simulink model "q_sip_lqr_mq3_ip01"  (Simulink 4.00)
settings: Solver=ode4  SolverMode=SingleTasking  StartTime=0.0  StopTime=9999  FixedStep=0.001  RelTol=1e-3  AbsTol=1e-6
values from neighbouring files (symbols this model uses):
  C = eye( 4 )    [d_ip01_2_sip_lqr.m]
  D = zeros( 4, 1 )    [d_ip01_2_sip_lqr.m]
undefined symbols (not defined in the file or in its folder): A, ALPHA_LIM_ENABLE, ALPHA_MAX, ALPHA_MIN, B, K, K_CABLE, K_PC, K_PP, simget, VMAX_DAC, VMAX_UPM, wcf, X_LIM_ENABLE, X_MAX, X_MIN, zetaf
libraries: qctools x6, simulink_extras x3
settings Model: LastModifiedBy=herve  LimitDataPoints=off  SimulationMode=external  RTWSystemTargetFile=wincon.tlc  RTWTemplateMakefile=nt_msvc.tmf  RTWMakeCommand=make_wc  ExtModeMexFile=wc_comm  ExtModeArmWhenConnect=off  OptimizeBlockIOStorage=off

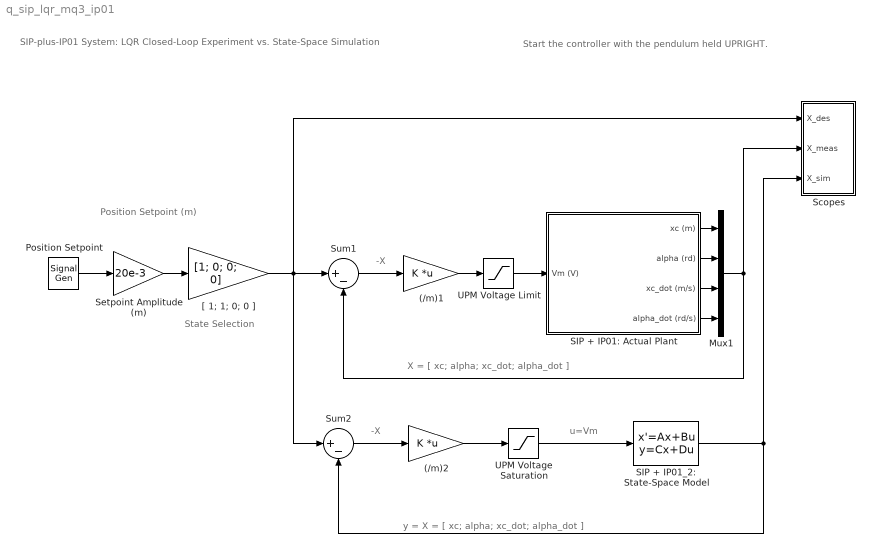
== system q_sip_lqr_mq3_ip01 ==
  note: SIP-plus-IP01 System: LQR Closed-Loop
      | Experiment vs. State-Space Simulation
  note: u=Vm
  note: X = [ xc; alpha; xc_dot; alpha_dot ]
  note: -X
  note: -X
  note: State Selection
  note: Start the controller with the pendulum held UPRIGHT.
  note: Position Setpoint (m)
  note: y = X = [ xc; alpha; xc_dot; alpha_dot ]
  (/m)1 : Gain  Gain=K  Multiplication=Matrix(K*u)  SaturateOnIntegerOverflow=on
  (/m)2 : Gain  Gain=K  Multiplication=Matrix(K*u)  SaturateOnIntegerOverflow=on
  Mux1 : Mux  Inputs=4
  Position Setpoint : SignalGenerator  WaveForm=square  Amplitude=1  Frequency=0.2  Units=Hertz
  SIP + IP01: Actual Plant : Subsystem
      settings: RTWFcnNameOpts=Auto  RTWFileNameOpts=Auto
  SIP + IP01_2: State-Space Model : StateSpace  A=A  B=B  C=C  D=D  X0=0  AbsoluteTolerance=auto  Realization=auto
  Scopes : Subsystem
      settings: RTWFcnNameOpts=Auto  RTWFileNameOpts=Auto
  Setpoint Amplitude (m) : Gain  Gain=20e-3  Multiplication=Element-wise(K.*u)  SaturateOnIntegerOverflow=on
  Sum1 : Sum  Inputs=|+-  SaturateOnIntegerOverflow=on
  Sum2 : Sum  Inputs=|+-  SaturateOnIntegerOverflow=on
  UPM Voltage Limit : Saturate  UpperLimit=VMAX_UPM  LowerLimit=- VMAX_UPM  LinearizeAsGain=on
  UPM Voltage Saturation : Saturate  UpperLimit=VMAX_UPM  LowerLimit=- VMAX_UPM  LinearizeAsGain=on
  "[ 1; 1; 0; 0 ]" : Gain  Gain=[1; 0; 0; 0]  Multiplication=Element-wise(K.*u)  SaturateOnIntegerOverflow=on
  wires:
  UPM Voltage Limit/1 -> SIP + IP01: Actual Plant/1(Vm (V))
  SIP + IP01: Actual Plant/1(xc (m)) -> Mux1/1
  (/m)1/1 -> UPM Voltage Limit/1
  SIP + IP01: Actual Plant/2(alpha (rd)) -> Mux1/2
  SIP + IP01: Actual Plant/4(alpha_dot (rd/s)) -> Mux1/4
  UPM Voltage Saturation/1 -> SIP + IP01_2: State-Space Model/1
  (/m)2/1 -> UPM Voltage Saturation/1
  Sum2/1 -> (/m)2/1
  Sum1/1 -> (/m)1/1
  "[ 1; 1; 0; 0 ]"/1 -> Sum1/1, Sum2/1, Scopes/1(X_des)
  Mux1/1 -> Sum1/2, Scopes/2(X_meas)
  SIP + IP01_2: State-Space Model/1 -> Sum2/2, Scopes/3(X_sim)
  Setpoint Amplitude (m)/1 -> "[ 1; 1; 0; 0 ]"/1
  SIP + IP01: Actual Plant/3(xc_dot (m/s)) -> Mux1/3
  Position Setpoint/1 -> Setpoint Amplitude (m)/1

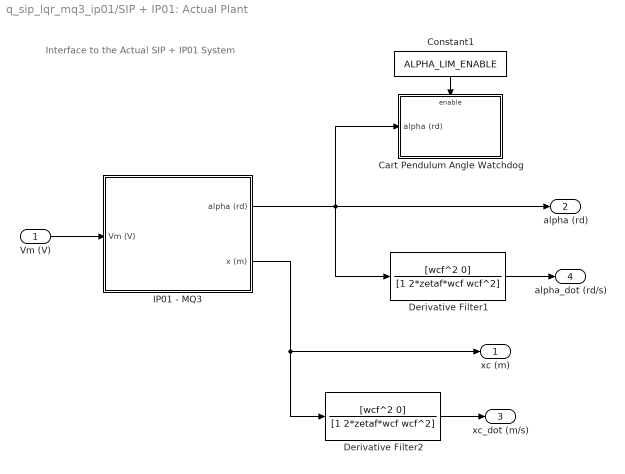
== system q_sip_lqr_mq3_ip01/SIP + IP01: Actual Plant ==
  note: Interface to the Actual
      | SIP + IP01 System
  Vm (V) : Inport  Port=1  LatchInput=off
  Cart Pendulum Angle Watchdog : Subsystem  TreatAsAtomicUnit=on
      settings: RTWFcnNameOpts=Auto  RTWFileNameOpts=Auto
  Constant1 : Constant  Orientation=down  Value=ALPHA_LIM_ENABLE
  Derivative Filter1 : TransferFcn  Numerator=[wcf^2 0]  Denominator=[1 2*zetaf*wcf wcf^2]  AbsoluteTolerance=auto  Realization=auto
  Derivative Filter2 : TransferFcn  Numerator=[wcf^2 0]  Denominator=[1 2*zetaf*wcf wcf^2]  AbsoluteTolerance=auto  Realization=auto
  IP01 - MQ3 : Subsystem
      settings: RTWFcnNameOpts=Auto  RTWFileNameOpts=Auto
  xc (m) : Outport  Port=1  InitialOutput=0
  alpha (rd) : Outport  Port=2  InitialOutput=0
  xc_dot (m/s) : Outport  Port=3  InitialOutput=0
  alpha_dot (rd/s) : Outport  Port=4  InitialOutput=0
  wires:
  Vm (V)/1 -> IP01 - MQ3/1(Vm (V))
  IP01 - MQ3/2(x (m)) -> Derivative Filter2/1, xc (m)/1
  IP01 - MQ3/1(alpha (rd)) -> Derivative Filter1/1, alpha (rd)/1, Cart Pendulum Angle Watchdog/1(alpha (rd))
  Derivative Filter2/1 -> xc_dot (m/s)/1
  Derivative Filter1/1 -> alpha_dot (rd/s)/1
  Constant1/1 -> Cart Pendulum Angle Watchdog/Enable

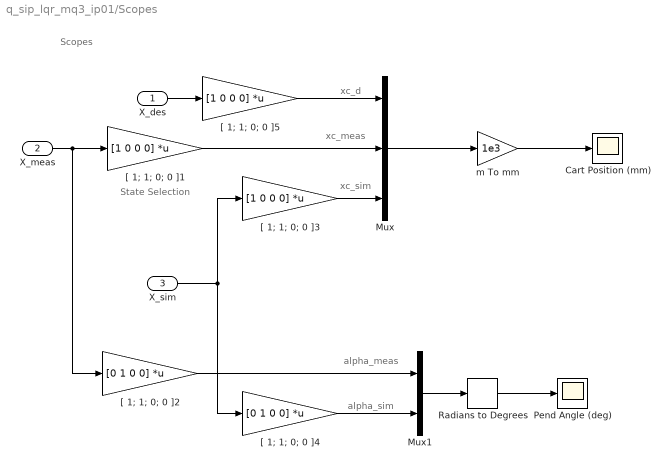
== system q_sip_lqr_mq3_ip01/Scopes ==
  note: xc_meas
  note: State Selection
  note: alpha_meas
  note: alpha_sim
  note: xc_sim
  note: xc_d
  note: Scopes
  X_des : Inport  Port=1  LatchInput=off
  X_meas : Inport  Port=2  LatchInput=off
  X_sim : Inport  Port=3  LatchInput=off
  Cart Position (mm) : Scope
      settings: TickLabels=on  TimeRange=1.000000  YMin=-250  YMax=250  SaveToWorkspace=off  DataFormat=Array  LimitDataPoints=on  MaxDataPoints=5000
  Mux : Mux  Inputs=3
  Mux1 : Mux  Inputs=2
  Pend Angle (deg) : Scope
      settings: TickLabels=on  TimeRange=1.000000  YMin=-250  YMax=250  SaveToWorkspace=off  SaveName=ScopeData  DataFormat=Array  LimitDataPoints=on  MaxDataPoints=5000
  Radians to Degrees : simulink_extras/Transformations/Radians to Degrees
  "[ 1; 1; 0; 0 ]1" : Gain  Gain=[1 0 0 0]  Multiplication=Matrix(K*u)  SaturateOnIntegerOverflow=on
  "[ 1; 1; 0; 0 ]2" : Gain  Gain=[0 1 0 0]  Multiplication=Matrix(K*u)  SaturateOnIntegerOverflow=on
  "[ 1; 1; 0; 0 ]3" : Gain  Gain=[1 0 0 0]  Multiplication=Matrix(K*u)  SaturateOnIntegerOverflow=on
  "[ 1; 1; 0; 0 ]4" : Gain  Gain=[0 1 0 0]  Multiplication=Matrix(K*u)  SaturateOnIntegerOverflow=on
  "[ 1; 1; 0; 0 ]5" : Gain  Gain=[1 0 0 0]  Multiplication=Matrix(K*u)  SaturateOnIntegerOverflow=on
  m To mm : Gain  Gain=1e3  Multiplication=Element-wise(K.*u)  SaturateOnIntegerOverflow=on
  wires:
  Mux/1 -> m To mm/1
  m To mm/1 -> Cart Position (mm)/1
  "[ 1; 1; 0; 0 ]1"/1 -> Mux/2
  X_des/1 -> "[ 1; 1; 0; 0 ]5"/1
  X_meas/1 -> "[ 1; 1; 0; 0 ]1"/1, "[ 1; 1; 0; 0 ]2"/1
  Mux1/1 -> Radians to Degrees/1
  Radians to Degrees/1 -> Pend Angle (deg)/1
  X_sim/1 -> "[ 1; 1; 0; 0 ]3"/1, "[ 1; 1; 0; 0 ]4"/1
  "[ 1; 1; 0; 0 ]3"/1 -> Mux/3
  "[ 1; 1; 0; 0 ]5"/1 -> Mux/1
  "[ 1; 1; 0; 0 ]2"/1 -> Mux1/1
  "[ 1; 1; 0; 0 ]4"/1 -> Mux1/2

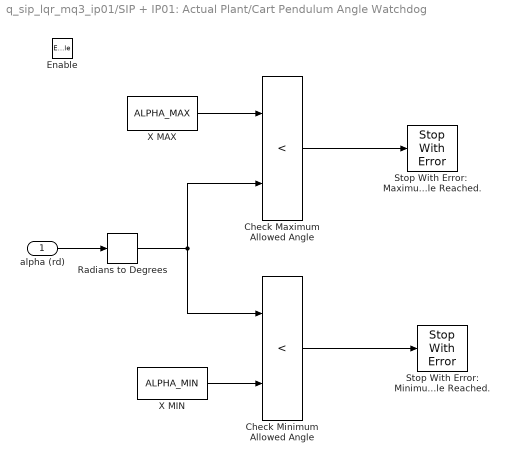
== system q_sip_lqr_mq3_ip01/SIP + IP01: Actual Plant/Cart Pendulum Angle Watchdog ==
  alpha (rd) : Inport  Port=1  LatchInput=off
  Enable : EnablePort
  Check Maximum Allowed Angle : RelationalOperator  Operator=<
  Check Minimum Allowed Angle : RelationalOperator  Operator=<
  Radians to Degrees : simulink_extras/Transformations/Radians to Degrees
  Stop With Error: Minimum Angle Reached. : qctools/Extra Sinks/Stop With Error  errMsg=Minimum Angle Limit Reached.
  Stop With Error:  Maximum Angle Reached. : qctools/Extra Sinks/Stop With Error  errMsg=Maximum Angle Limit Reached.
  X MAX : Constant  Value=ALPHA_MAX
  X MIN : Constant  Value=ALPHA_MIN
  wires:
  X MAX/1 -> Check Maximum Allowed Angle/1
  Check Minimum Allowed Angle/1 -> Stop With Error: Minimum Angle Reached./1
  X MIN/1 -> Check Minimum Allowed Angle/2
  alpha (rd)/1 -> Radians to Degrees/1
  Check Maximum Allowed Angle/1 -> Stop With Error:  Maximum Angle Reached./1
  Radians to Degrees/1 -> Check Maximum Allowed Angle/2, Check Minimum Allowed Angle/1

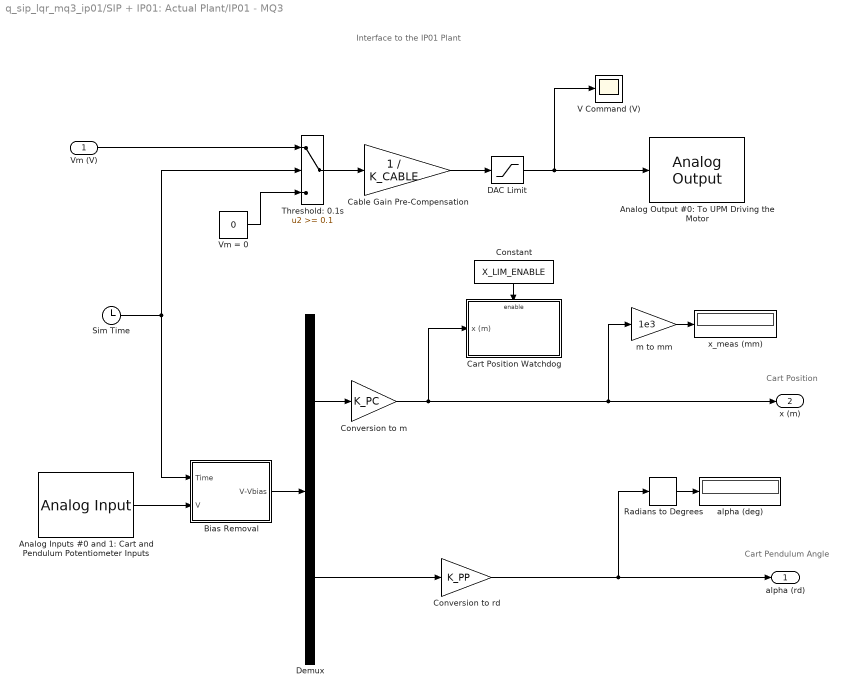
== system q_sip_lqr_mq3_ip01/SIP + IP01: Actual Plant/IP01 - MQ3 ==
  note: Cart Position
  note: Cart Pendulum Angle
  note: Interface to the IP01 Plant
  Vm (V) : Inport  Port=1  LatchInput=off
  "Analog Inputs #0 and 1: Cart and Pendulum Potentiometer Inputs " : qctools/Quanser Consulting MQ3 Series/Analog Input  baseAddr=0x320  channels=[0 1]  sampleTime=simget(bdroot,'FixedStep')  simulationInput=off
  Analog Output #0: To UPM Driving the Motor : qctools/Quanser Consulting MQ3 Series/Analog Output  baseAddr=0x320  channels=0  initialOutputs=0  finalOutputs=0  sampleTime=-1  simulationOutput=off
  Bias Removal : Subsystem  TreatAsAtomicUnit=on
      settings: RTWFcnNameOpts=Auto  RTWFileNameOpts=Auto
  Cable Gain Pre-Compensation : Gain  Gain=1 / K_CABLE  Multiplication=Element-wise(K.*u)  SaturateOnIntegerOverflow=on
  Cart Position Watchdog : Subsystem  TreatAsAtomicUnit=on
      settings: RTWFcnNameOpts=Auto  RTWFileNameOpts=Auto
  Constant : Constant  Orientation=down  Value=X_LIM_ENABLE
  Conversion to m : Gain  Gain=K_PC  Multiplication=Element-wise(K.*u)  SaturateOnIntegerOverflow=on
  Conversion to rd : Gain  Gain=K_PP  Multiplication=Element-wise(K.*u)  SaturateOnIntegerOverflow=on
  DAC Limit : Saturate  UpperLimit=VMAX_DAC  LowerLimit=- VMAX_DAC  LinearizeAsGain=on
  Demux : Demux  Outputs=2  BusSelectionMode=off
  Radians to Degrees : simulink_extras/Transformations/Radians to Degrees
  Sim Time : Clock
      settings: DisplayTime=off
  Threshold: 0.1s : Switch  Threshold=0.1
  V Command (V) : Scope
      settings: TickLabels=on  TimeRange=1.000000  YMin=-1  YMax=1  SaveToWorkspace=off  SaveName=ScopeData3  DataFormat=Array  LimitDataPoints=on  MaxDataPoints=5000
  Vm = 0 : Constant  Value=0
  alpha (deg) : Display
      settings: Format=short
  m to mm : Gain  Gain=1e3  Multiplication=Element-wise(K.*u)  SaturateOnIntegerOverflow=on
  x_meas (mm) : Display
      settings: Format=short
  alpha (rd) : Outport  Port=1  InitialOutput=0
  x (m) : Outport  Port=2  InitialOutput=0
  wires:
  Demux/1 -> Conversion to m/1
  Demux/2 -> Conversion to rd/1
  "Analog Inputs #0 and 1: Cart and Pendulum Potentiometer Inputs "/1 -> Bias Removal/2(V)
  DAC Limit/1 -> V Command (V)/1, Analog Output #0: To UPM Driving the Motor/1
  Constant/1 -> Cart Position Watchdog/Enable
  Conversion to rd/1 -> alpha (rd)/1, Radians to Degrees/1
  Radians to Degrees/1 -> alpha (deg)/1
  m to mm/1 -> x_meas (mm)/1
  Cable Gain Pre-Compensation/1 -> DAC Limit/1
  Conversion to m/1 -> m to mm/1, x (m)/1, Cart Position Watchdog/1(x (m))
  Bias Removal/1(V-Vbias) -> Demux/1
  Sim Time/1 -> Threshold: 0.1s/2, Bias Removal/1(Time)
  Vm = 0/1 -> Threshold: 0.1s/3
  Vm (V)/1 -> Threshold: 0.1s/1
  Threshold: 0.1s/1 -> Cable Gain Pre-Compensation/1

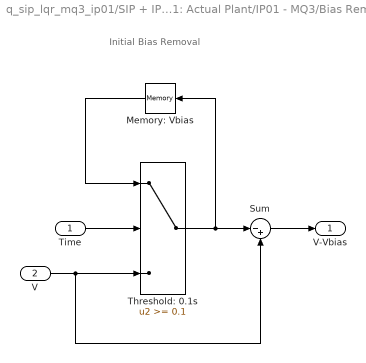
== system q_sip_lqr_mq3_ip01/SIP + IP01: Actual Plant/IP01 - MQ3/Bias Removal ==
  note: Initial Bias Removal
  Time : Inport  Port=1  LatchInput=off
  V : Inport  Port=2  LatchInput=off
  Memory: Vbias : Memory  Orientation=left  X0=0  InheritSampleTime=off
      settings: RTWStateStorageClass=Auto
  Sum : Sum  Inputs=|-+  SaturateOnIntegerOverflow=on
  Threshold: 0.1s : Switch  Threshold=0.1
  V-Vbias : Outport  Port=1
  wires:
  V/1 -> Threshold: 0.1s/3, Sum/2
  Memory: Vbias/1 -> Threshold: 0.1s/1
  Threshold: 0.1s/1 -> Memory: Vbias/1, Sum/1
  Sum/1 -> V-Vbias/1
  Time/1 -> Threshold: 0.1s/2

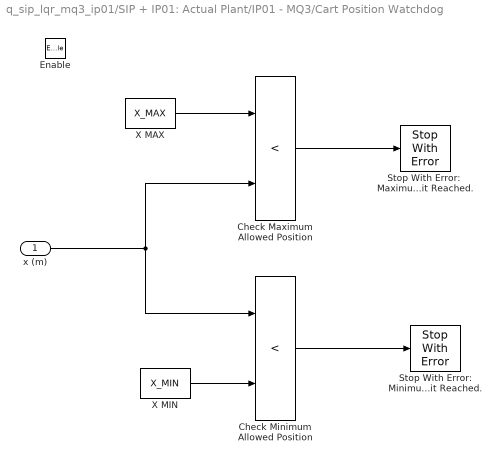
== system q_sip_lqr_mq3_ip01/SIP + IP01: Actual Plant/IP01 - MQ3/Cart Position Watchdog ==
  x (m) : Inport  Port=1  LatchInput=off
  Enable : EnablePort
  Check Maximum Allowed Position : RelationalOperator  Operator=<
  Check Minimum Allowed Position : RelationalOperator  Operator=<
  Stop With Error: Minimum Limit Reached. : qctools/Extra Sinks/Stop With Error  errMsg=Minimum Position Limit reached.
  Stop With Error:  Maximum Limit Reached. : qctools/Extra Sinks/Stop With Error  errMsg=Maximum Position Limit reached.
  X MAX : Constant  Value=X_MAX
  X MIN : Constant  Value=X_MIN
  wires:
  X MAX/1 -> Check Maximum Allowed Position/1
  Check Minimum Allowed Position/1 -> Stop With Error: Minimum Limit Reached./1
  X MIN/1 -> Check Minimum Allowed Position/2
  x (m)/1 -> Check Maximum Allowed Position/2, Check Minimum Allowed Position/1
  Check Maximum Allowed Position/1 -> Stop With Error:  Maximum Limit Reached./1
